simulink model "PI_Level_Control"  (R2024b)
settings: Solver=VariableStepAuto  StartTime=0.0  StopTime=1000  RelTol=1e-3
values from neighbouring files (symbols this model uses):
  C = 6.8    [Arduino_Control_Script.m]    (also in PI_Level_Control_Script.m)
  k = 0.032    [Arduino_Control_Script.m]    (also in PI_Level_Control_Script.m)
  k1 = 0.624    [Arduino_Control_Script.m]    (also in PI_Level_Control_Script.m)
  k11 = k2^2+4*(k-k3)*k1    (= 0.0815946)    [Arduino_Control_Script.m]    (also in PI_Level_Control_Script.m)
  k12 = 8*(k-k3)    (= 0.2608)    [Arduino_Control_Script.m]    (also in PI_Level_Control_Script.m)
  k13 = 2*(k-k3)    (= 0.0652)    [Arduino_Control_Script.m]    (also in PI_Level_Control_Script.m)
  k2 = -0.015    [Arduino_Control_Script.m]    (also in PI_Level_Control_Script.m)
  k3 = -0.0006    [Arduino_Control_Script.m]    (also in PI_Level_Control_Script.m)
  keta = 8*10^-5    (= 8e-05)    [Arduino_Control_Script.m]    (also in PI_Level_Control_Script.m)
libraries: slpidlib x20
(part 2 of 3)

== system PI_Level_Control/Model Proces ==
  ua : Inport
  Amplificator : Subsystem
  Curent Rotoric : Subsystem
  Filtru : Subsystem
  Motor : Subsystem
  Pompa : Subsystem
  Randament Pompa : Subsystem
  Rezervor : Subsystem
  h : Outport
  q : Outport  Port=2
  wires:
  Randament Pompa/1(eta) -> Curent Rotoric/3(eta)
  Rezervor/1(h) -> h/1, Curent Rotoric/1(h), Pompa/2(h)
  Curent Rotoric/1(im) -> Motor/2(im)
  Amplificator/1(um) -> Motor/1(um), Randament Pompa/2(um), Curent Rotoric/4(um)
  ua/1 -> Amplificator/1(ua)
  Filtru/1(q_f) -> Rezervor/1(q), Curent Rotoric/2(q), q/1, Randament Pompa/1(q)
  Pompa/1(q) -> Filtru/1(q)
  Motor/1(kn) -> Pompa/1(kn)

== system PI_Level_Control/Model Proces Nivel ==
  ua : Inport
  Amplificator : Subsystem
  Curent Rotoric : Subsystem
  Filtru : Subsystem
  Motor : Subsystem
  Pompa : Subsystem
  Randament Pompa : Subsystem
  Rezervor : Subsystem
  h : Outport
  q : Outport  Port=2
  wires:
  Randament Pompa/1(eta) -> Curent Rotoric/3(eta)
  Rezervor/1(h) -> h/1, Curent Rotoric/1(h), Pompa/2(h)
  Curent Rotoric/1(im) -> Motor/2(im)
  Amplificator/1(um) -> Motor/1(um), Randament Pompa/2(um), Curent Rotoric/4(um)
  ua/1 -> Amplificator/1(ua)
  Filtru/1(q_f) -> Rezervor/1(q), Curent Rotoric/2(q), q/1, Randament Pompa/1(q)
  Pompa/1(q) -> Filtru/1(q)
  Motor/1(kn) -> Pompa/1(kn)

== system PI_Level_Control/Model Proces Nivel1 ==
  ua : Inport
  Amplificator : Subsystem
  Curent Rotoric : Subsystem
  Filtru : Subsystem
  Motor : Subsystem
  Pompa : Subsystem
  Randament Pompa : Subsystem
  Rezervor : Subsystem
  h : Outport
  q : Outport  Port=2
  wires:
  Randament Pompa/1(eta) -> Curent Rotoric/3(eta)
  Rezervor/1(h) -> h/1, Curent Rotoric/1(h), Pompa/2(h)
  Curent Rotoric/1(im) -> Motor/2(im)
  Amplificator/1(um) -> Motor/1(um), Randament Pompa/2(um), Curent Rotoric/4(um)
  ua/1 -> Amplificator/1(ua)
  Filtru/1(q_f) -> Rezervor/1(q), Curent Rotoric/2(q), q/1, Randament Pompa/1(q)
  Pompa/1(q) -> Filtru/1(q)
  Motor/1(kn) -> Pompa/1(kn)

== system PI_Level_Control/Model Proces Nivel2 ==
  ua : Inport
  Amplificator : Subsystem
  Curent Rotoric : Subsystem
  Filtru : Subsystem
  Motor : Subsystem
  Pompa : Subsystem
  Randament Pompa : Subsystem
  Rezervor : Subsystem
  h : Outport
  q : Outport  Port=2
  wires:
  Randament Pompa/1(eta) -> Curent Rotoric/3(eta)
  Rezervor/1(h) -> h/1, Curent Rotoric/1(h), Pompa/2(h)
  Curent Rotoric/1(im) -> Motor/2(im)
  Amplificator/1(um) -> Motor/1(um), Randament Pompa/2(um), Curent Rotoric/4(um)
  ua/1 -> Amplificator/1(ua)
  Filtru/1(q_f) -> Rezervor/1(q), Curent Rotoric/2(q), q/1, Randament Pompa/1(q)
  Pompa/1(q) -> Filtru/1(q)
  Motor/1(kn) -> Pompa/1(kn)

== system PI_Level_Control/Model Proces Nivel3 ==
  ua : Inport
  Amplificator : Subsystem
  Curent Rotoric : Subsystem
  Filtru : Subsystem
  Motor : Subsystem
  Pompa : Subsystem
  Randament Pompa : Subsystem
  Rezervor : Subsystem
  h : Outport
  q : Outport  Port=2
  wires:
  Randament Pompa/1(eta) -> Curent Rotoric/3(eta)
  Rezervor/1(h) -> h/1, Curent Rotoric/1(h), Pompa/2(h)
  Curent Rotoric/1(im) -> Motor/2(im)
  Amplificator/1(um) -> Motor/1(um), Randament Pompa/2(um), Curent Rotoric/4(um)
  ua/1 -> Amplificator/1(ua)
  Filtru/1(q_f) -> Rezervor/1(q), Curent Rotoric/2(q), q/1, Randament Pompa/1(q)
  Pompa/1(q) -> Filtru/1(q)
  Motor/1(kn) -> Pompa/1(kn)

== system PI_Level_Control/Model Proces1 ==
  ua : Inport
  Amplificator : Subsystem
  Curent Rotoric : Subsystem
  Filtru : Subsystem
  Motor : Subsystem
  Pompa : Subsystem
  Randament Pompa : Subsystem
  Rezervor : Subsystem
  h : Outport
  wires:
  Randament Pompa/1(eta) -> Curent Rotoric/3(eta)
  Rezervor/1(h) -> h/1, Pompa/2(h), Curent Rotoric/1(h)
  Curent Rotoric/1(im) -> Motor/2(im)
  Amplificator/1(um) -> Motor/1(um), Randament Pompa/2(um), Curent Rotoric/4(um)
  ua/1 -> Amplificator/1(ua)
  Filtru/1(q_f) -> Rezervor/1(q), Randament Pompa/1(q), Curent Rotoric/2(q)
  Pompa/1(q) -> Filtru/1(q)
  Motor/1(kn) -> Pompa/1(kn)

== system PI_Level_Control/Model Proces10 ==
  ua : Inport
  Amplificator : Subsystem
  Curent Rotoric : Subsystem
  Filtru : Subsystem
  Motor : Subsystem
  Pompa cu perturbatie reala : Subsystem
  Randament Pompa : Subsystem
  Rezervor : Subsystem
  Step : Step  Time=250  After=0.1*k  SampleTime=0
  h : Outport
  qi : Outport  Port=2
  wires:
  Randament Pompa/1(eta) -> Curent Rotoric/3(eta)
  Rezervor/1(h) -> Pompa cu perturbatie reala/3(h), Curent Rotoric/1(h), h/1
  Curent Rotoric/1(im) -> Motor/2(im)
  Amplificator/1(um) -> Motor/1(um), Randament Pompa/2(um), Curent Rotoric/4(um)
  ua/1 -> Amplificator/1(ua)
  Pompa cu perturbatie reala/1(q) -> Filtru/1(q)
  Motor/1(kn) -> Pompa cu perturbatie reala/1(kn)
  Filtru/1(q_f) -> Rezervor/1(q), Randament Pompa/1(q), qi/1, Curent Rotoric/2(q)
  Step/1 -> Pompa cu perturbatie reala/2(perturbatie k)

== system PI_Level_Control/Model Proces11 ==
  ua : Inport
  Amplificator : Subsystem
  Curent Rotoric : Subsystem
  Filtru : Subsystem
  Motor : Subsystem
  Pompa cu perturbatie reala : Subsystem
  Randament Pompa : Subsystem
  Rezervor1 : Subsystem
  Step : Step  Time=400  After=0.1*k  SampleTime=0
  h : Outport
  qi : Outport  Port=2
  wires:
  Randament Pompa/1(eta) -> Curent Rotoric/3(eta)
  Rezervor1/1(h) -> Pompa cu perturbatie reala/3(h), Curent Rotoric/1(h), h/1
  Curent Rotoric/1(im) -> Motor/2(im)
  Amplificator/1(um) -> Motor/1(um), Randament Pompa/2(um), Curent Rotoric/4(um)
  ua/1 -> Amplificator/1(ua)
  Pompa cu perturbatie reala/1(q) -> Filtru/1(q)
  Motor/1(kn) -> Pompa cu perturbatie reala/1(kn)
  Filtru/1(q_f) -> Rezervor1/1(q), Randament Pompa/1(q), qi/1, Curent Rotoric/2(q)
  Step/1 -> Pompa cu perturbatie reala/2(perturbatie k)

== system PI_Level_Control/Model Proces12 ==
  ua : Inport
  Amplificator : Subsystem
  Curent Rotoric : Subsystem
  Filtru : Subsystem
  Motor : Subsystem
  Pompa cu perturbatie reala : Subsystem
  Randament Pompa : Subsystem
  Rezervor : Subsystem
  perturbatie k : Step  Time=300  After=0.1*k  SampleTime=0
  h : Outport
  qi : Outport  Port=2
  perturbatie : Outport  Port=3
  wires:
  Randament Pompa/1(eta) -> Curent Rotoric/3(eta)
  Rezervor/1(h) -> Pompa cu perturbatie reala/3(h), Curent Rotoric/1(h), h/1
  Curent Rotoric/1(im) -> Motor/2(im)
  Amplificator/1(um) -> Motor/1(um), Randament Pompa/2(um), Curent Rotoric/4(um)
  ua/1 -> Amplificator/1(ua)
  Pompa cu perturbatie reala/1(q) -> Filtru/1(q)
  Motor/1(kn) -> Pompa cu perturbatie reala/1(kn)
  Filtru/1(q_f) -> Randament Pompa/1(q), Curent Rotoric/2(q), qi/1, Rezervor/1(q)
  perturbatie k/1 -> Pompa cu perturbatie reala/2(perturbatie k)
  Rezervor/2(perturbatie) -> perturbatie/1

== system PI_Level_Control/Model Proces13 ==
  ua : Inport
  Amplificator : Subsystem
  Curent Rotoric : Subsystem
  Filtru : Subsystem
  Motor : Subsystem
  Pompa cu perturbatie reala : Subsystem
  Randament Pompa : Subsystem
  Rezervor : Subsystem
  perturbatie k : Step  Time=450  After=0.1*k  SampleTime=0
  h : Outport
  qi : Outport  Port=2
  perturbatie : Outport  Port=3
  wires:
  Randament Pompa/1(eta) -> Curent Rotoric/3(eta)
  Rezervor/1(h) -> Pompa cu perturbatie reala/3(h), Curent Rotoric/1(h), h/1
  Curent Rotoric/1(im) -> Motor/2(im)
  Amplificator/1(um) -> Motor/1(um), Randament Pompa/2(um), Curent Rotoric/4(um)
  ua/1 -> Amplificator/1(ua)
  Pompa cu perturbatie reala/1(q) -> Filtru/1(q)
  Motor/1(kn) -> Pompa cu perturbatie reala/1(kn)
  Filtru/1(q_f) -> Randament Pompa/1(q), Curent Rotoric/2(q), qi/1, Rezervor/1(q)
  perturbatie k/1 -> Pompa cu perturbatie reala/2(perturbatie k)
  Rezervor/2(perturbatie) -> perturbatie/1

== system PI_Level_Control/Model Proces2 ==
  ua : Inport
  Amplificator : Subsystem
  Curent Rotoric : Subsystem
  Filtru : Subsystem
  Motor : Subsystem
  Pompa : Subsystem
  Randament Pompa : Subsystem
  Rezervor : Subsystem
  h : Outport
  wires:
  Randament Pompa/1(eta) -> Curent Rotoric/3(eta)
  Rezervor/1(h) -> h/1, Pompa/2(h), Curent Rotoric/1(h)
  Curent Rotoric/1(im) -> Motor/2(im)
  Amplificator/1(um) -> Motor/1(um), Randament Pompa/2(um), Curent Rotoric/4(um)
  ua/1 -> Amplificator/1(ua)
  Filtru/1(q_f) -> Rezervor/1(q), Randament Pompa/1(q), Curent Rotoric/2(q)
  Pompa/1(q) -> Filtru/1(q)
  Motor/1(kn) -> Pompa/1(kn)

== system PI_Level_Control/Model Proces3 ==
  ua : Inport
  Amplificator : Subsystem
  Curent Rotoric : Subsystem
  Delta qe grafic : Scope
  Detla qe : Display
  Filtru : Subsystem
  Motor : Subsystem
  Pompa : Subsystem
  Randament Pompa : Subsystem
  Rezervor : Subsystem
  h : Outport
  wires:
  Randament Pompa/1(eta) -> Curent Rotoric/3(eta)
  Rezervor/1(h) -> Curent Rotoric/1(h), Pompa/2(h), h/1
  Curent Rotoric/1(im) -> Motor/2(im)
  Amplificator/1(um) -> Motor/1(um), Randament Pompa/2(um), Curent Rotoric/4(um)
  ua/1 -> Amplificator/1(ua)
  Filtru/1(q_f) -> Randament Pompa/1(q), Curent Rotoric/2(q), Rezervor/1(q)
  Pompa/1(q) -> Filtru/1(q)
  Motor/1(kn) -> Pompa/1(kn)
  Rezervor/2(perturbatie) -> Delta qe grafic/1, Detla qe/1

== system PI_Level_Control/Model Proces4 ==
  ua : Inport
  Amplificator : Subsystem
  Curent Rotoric : Subsystem
  Delta qe grafic : Scope
  Detla qe : Display
  Filtru : Subsystem
  Motor : Subsystem
  Pompa : Subsystem
  Randament Pompa : Subsystem
  Rezervor : Subsystem
  h : Outport
  wires:
  Randament Pompa/1(eta) -> Curent Rotoric/3(eta)
  Rezervor/1(h) -> Curent Rotoric/1(h), Pompa/2(h), h/1
  Curent Rotoric/1(im) -> Motor/2(im)
  Amplificator/1(um) -> Motor/1(um), Randament Pompa/2(um), Curent Rotoric/4(um)
  ua/1 -> Amplificator/1(ua)
  Filtru/1(q_f) -> Randament Pompa/1(q), Curent Rotoric/2(q), Rezervor/1(q)
  Pompa/1(q) -> Filtru/1(q)
  Motor/1(kn) -> Pompa/1(kn)
  Rezervor/2(perturbatie) -> Delta qe grafic/1, Detla qe/1

== system PI_Level_Control/Model Proces5 ==
  ua : Inport
  Amplificator : Subsystem
  Curent Rotoric : Subsystem
  Filtru : Subsystem
  Motor : Subsystem
  Perturbatie 10%k : Step  Time=250  After=k*0.1  SampleTime=0
  Pompa cu perturbatie reala : Subsystem
  Randament Pompa : Subsystem
  Rezervor : Subsystem
  h : Outport
  wires:
  Randament Pompa/1(eta) -> Curent Rotoric/3(eta)
  Rezervor/1(h) -> h/1, Pompa cu perturbatie reala/3(h), Curent Rotoric/1(h)
  Curent Rotoric/1(im) -> Motor/2(im)
  Amplificator/1(um) -> Motor/1(um), Randament Pompa/2(um), Curent Rotoric/4(um)
  ua/1 -> Amplificator/1(ua)
  Filtru/1(q_f) -> Rezervor/1(q), Randament Pompa/1(q), Curent Rotoric/2(q)
  Pompa cu perturbatie reala/1(q) -> Filtru/1(q)
  Motor/1(kn) -> Pompa cu perturbatie reala/1(kn)
  Perturbatie 10%k/1 -> Pompa cu perturbatie reala/2(perturbatie k)

== system PI_Level_Control/Model Proces6 ==
  ua : Inport
  Amplificator : Subsystem
  Curent Rotoric : Subsystem
  Filtru : Subsystem
  Motor : Subsystem
  Perturbatie 10%k : Step  Time=250  After=k*0.1  SampleTime=0
  Pompa cu perturbatie reala : Subsystem
  Randament Pompa : Subsystem
  Rezervor1 : Subsystem
  h : Outport
  wires:
  Randament Pompa/1(eta) -> Curent Rotoric/3(eta)
  Rezervor1/1(h) -> h/1, Pompa cu perturbatie reala/3(h), Curent Rotoric/1(h)
  Curent Rotoric/1(im) -> Motor/2(im)
  Amplificator/1(um) -> Motor/1(um), Randament Pompa/2(um), Curent Rotoric/4(um)
  ua/1 -> Amplificator/1(ua)
  Filtru/1(q_f) -> Rezervor1/1(q), Randament Pompa/1(q), Curent Rotoric/2(q)
  Pompa cu perturbatie reala/1(q) -> Filtru/1(q)
  Motor/1(kn) -> Pompa cu perturbatie reala/1(kn)
  Perturbatie 10%k/1 -> Pompa cu perturbatie reala/2(perturbatie k)

== system PI_Level_Control/Model Proces7 ==
  ua : Inport
  Amplificator : Subsystem
  Curent Rotoric : Subsystem
  Filtru : Subsystem
  Motor : Subsystem
  Pompa : Subsystem
  Randament Pompa : Subsystem
  Rezervor : Subsystem
  h : Outport
  perturbatie delta qe : Outport  Port=2
  wires:
  Randament Pompa/1(eta) -> Curent Rotoric/3(eta)
  Rezervor/1(h) -> Curent Rotoric/1(h), Pompa/2(h), h/1
  Curent Rotoric/1(im) -> Motor/2(im)
  Amplificator/1(um) -> Motor/1(um), Randament Pompa/2(um), Curent Rotoric/4(um)
  ua/1 -> Amplificator/1(ua)
  Filtru/1(q_f) -> Randament Pompa/1(q), Curent Rotoric/2(q), Rezervor/1(q)
  Pompa/1(q) -> Filtru/1(q)
  Motor/1(kn) -> Pompa/1(kn)
  Rezervor/2(perturbatie) -> perturbatie delta qe/1

== system PI_Level_Control/Model Proces8 ==
  ua : Inport
  Amplificator : Subsystem
  Curent Rotoric : Subsystem
  Filtru : Subsystem
  Motor : Subsystem
  Pompa : Subsystem
  Randament Pompa : Subsystem
  Rezervor : Subsystem
  h : Outport
  perturbatie delta qe : Outport  Port=2
  wires:
  Randament Pompa/1(eta) -> Curent Rotoric/3(eta)
  Rezervor/1(h) -> Curent Rotoric/1(h), Pompa/2(h), h/1
  Curent Rotoric/1(im) -> Motor/2(im)
  Amplificator/1(um) -> Motor/1(um), Randament Pompa/2(um), Curent Rotoric/4(um)
  ua/1 -> Amplificator/1(ua)
  Filtru/1(q_f) -> Randament Pompa/1(q), Curent Rotoric/2(q), Rezervor/1(q)
  Pompa/1(q) -> Filtru/1(q)
  Motor/1(kn) -> Pompa/1(kn)
  Rezervor/2(perturbatie) -> perturbatie delta qe/1

== system PI_Level_Control/Model Proces9 ==
  ua : Inport
  Amplificator : Subsystem
  Curent Rotoric : Subsystem
  Filtru : Subsystem
  Motor : Subsystem
  Pompa : Subsystem
  Randament Pompa : Subsystem
  Rezervor : Subsystem
  h : Outport
  qi : Outport  Port=2
  wires:
  Randament Pompa/1(eta) -> Curent Rotoric/3(eta)
  Rezervor/1(h) -> Curent Rotoric/1(h), Pompa/2(h), h/1
  Curent Rotoric/1(im) -> Motor/2(im)
  Amplificator/1(um) -> Motor/1(um), Randament Pompa/2(um), Curent Rotoric/4(um)
  ua/1 -> Amplificator/1(ua)
  Pompa/1(q) -> Filtru/1(q)
  Motor/1(kn) -> Pompa/1(kn)
  Filtru/1(q_f) -> qi/1, Randament Pompa/1(q), Curent Rotoric/2(q), Rezervor/1(q)

== system PI_Level_Control/Model Proces/Amplificator ==
  ua : Inport
  Constant : Constant  Value=8.1
  Gain : Gain  Gain=2.2
  Gain1 : Gain  Gain=2.2
  Gain2 : Gain  Gain=5
  Saturation : Saturate  UpperLimit=22  LowerLimit=0
  Sum : Sum  Inputs=|+-
  Sum1 : Sum  Inputs=|++
  Switch : Switch  Threshold=8.1  SaturateOnIntegerOverflow=off  InputSameDT=off
  um : Outport
  wires:
  ua/1 -> Gain/1, Sum/1, Gain1/1, Switch/2
  Gain1/1 -> Sum1/1
  Gain/1 -> Switch/3
  Sum1/1 -> Switch/1
  Gain2/1 -> Sum1/2
  Constant/1 -> Sum/2
  Switch/1 -> Saturation/1
  Sum/1 -> Gain2/1
  Saturation/1 -> um/1

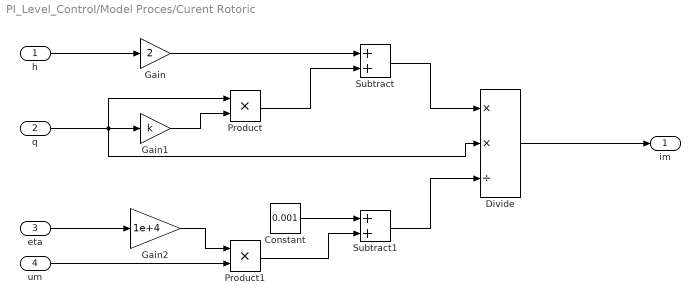
== system PI_Level_Control/Model Proces/Curent Rotoric ==
  h : Inport
  q : Inport  Port=2
  eta : Inport  Port=3
  um : Inport  Port=4
  Constant : Constant  Value=0.001
  Divide : Product  Inputs=**/
  Gain : Gain  Gain=2
  Gain1 : Gain  Gain=k
  Gain2 : Gain  Gain=1e+4
  Product : Product
  Product1 : Product
  Subtract : Sum
  Subtract1 : Sum
  im : Outport
  wires:
  Divide/1 -> im/1
  Subtract1/1 -> Divide/3
  Constant/1 -> Subtract1/1
  Gain2/1 -> Product1/1
  q/1 -> Divide/2, Product/1, Gain1/1
  Subtract/1 -> Divide/1
  Product/1 -> Subtract/2
  Gain/1 -> Subtract/1
  Gain1/1 -> Product/2
  Product1/1 -> Subtract1/2
  um/1 -> Product1/2
  h/1 -> Gain/1
  eta/1 -> Gain2/1

== system PI_Level_Control/Model Proces/Filtru ==
  q : Inport
  Integrator : Integrator  InitialCondition=29.18
  Sum : Sum  Inputs=|+-
  q_f : Outport
  wires:
  Sum/1 -> Integrator/1
  Integrator/1 -> q_f/1, Sum/2
  q/1 -> Sum/1

== system PI_Level_Control/Model Proces/Motor ==
  um : Inport
  im : Inport  Port=2
  Add : Sum  Inputs=+-
  Rm : Gain  Gain=3
  kn : Outport
  wires:
  Rm/1 -> Add/2
  um/1 -> Add/1
  im/1 -> Rm/1
  Add/1 -> kn/1

== system PI_Level_Control/Model Proces/Pompa ==
  kn : Inport
  h : Inport  Port=2
  Gain : Gain  Gain=k2
  Gain1 : Gain  Gain=k11
  Gain2 : Gain  Gain=k12
  Gain3 : Gain  Gain=1/k13
  Product : Product
  Sqrt : Sqrt
  Subtract : Sum  Inputs=+-
  Subtract1 : Sum
  q : Outport
  wires:
  Gain1/1 -> Subtract/1
  Gain2/1 -> Subtract/2
  Product/1 -> Gain1/1
  Gain/1 -> Subtract1/1
  kn/1 -> Product/2, Product/1, Gain/1
  Subtract/1 -> Sqrt/1
  Subtract1/1 -> Gain3/1
  Sqrt/1 -> Subtract1/2
  Gain3/1 -> q/1
  h/1 -> Gain2/1

== system PI_Level_Control/Model Proces/Randament Pompa ==
  q : Inport
  um : Inport  Port=2
  Gain : Gain  Gain=keta
  Product : Product
  eta : Outport
  wires:
  Gain/1 -> Product/2
  Product/1 -> eta/1
  q/1 -> Product/1
  um/1 -> Gain/1

== system PI_Level_Control/Model Proces/Rezervor ==
  q : Inport
  Fcn : Fcn  Expr=sqrt(u)*9
  Gain : Gain  Gain=1/332.5
  Integrator : Integrator  InitialCondition=10.51
  Sum : Sum  Inputs=|+-
  h : Outport
  wires:
  Gain/1 -> Integrator/1
  Fcn/1 -> Sum/2
  Integrator/1 -> h/1, Fcn/1
  Sum/1 -> Gain/1
  q/1 -> Sum/1

== system PI_Level_Control/Model Proces Nivel/Amplificator ==
  ua : Inport
  Constant : Constant  Value=8.1
  Gain : Gain  Gain=2.2
  Gain1 : Gain  Gain=2.2
  Gain2 : Gain  Gain=5
  Saturation : Saturate  UpperLimit=22  LowerLimit=0
  Sum : Sum  Inputs=|+-
  Sum1 : Sum  Inputs=|++
  Switch : Switch  Threshold=8.1  SaturateOnIntegerOverflow=off  InputSameDT=off
  um : Outport
  wires:
  ua/1 -> Gain/1, Sum/1, Gain1/1, Switch/2
  Gain1/1 -> Sum1/1
  Gain/1 -> Switch/3
  Sum1/1 -> Switch/1
  Gain2/1 -> Sum1/2
  Constant/1 -> Sum/2
  Switch/1 -> Saturation/1
  Sum/1 -> Gain2/1
  Saturation/1 -> um/1

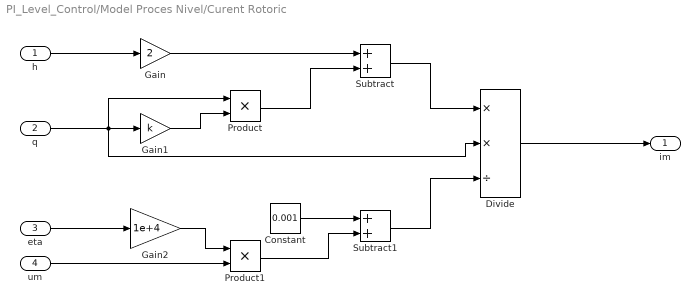
== system PI_Level_Control/Model Proces Nivel/Curent Rotoric ==
  h : Inport
  q : Inport  Port=2
  eta : Inport  Port=3
  um : Inport  Port=4
  Constant : Constant  Value=0.001
  Divide : Product  Inputs=**/
  Gain : Gain  Gain=2
  Gain1 : Gain  Gain=k
  Gain2 : Gain  Gain=1e+4
  Product : Product
  Product1 : Product
  Subtract : Sum
  Subtract1 : Sum
  im : Outport
  wires:
  Divide/1 -> im/1
  Subtract1/1 -> Divide/3
  Constant/1 -> Subtract1/1
  Gain2/1 -> Product1/1
  q/1 -> Divide/2, Product/1, Gain1/1
  Subtract/1 -> Divide/1
  Product/1 -> Subtract/2
  Gain/1 -> Subtract/1
  Gain1/1 -> Product/2
  Product1/1 -> Subtract1/2
  um/1 -> Product1/2
  h/1 -> Gain/1
  eta/1 -> Gain2/1

== system PI_Level_Control/Model Proces Nivel/Filtru ==
  q : Inport
  Integrator : Integrator  InitialCondition=27.3
  Sum : Sum  Inputs=|+-
  q_f : Outport
  wires:
  Sum/1 -> Integrator/1
  Integrator/1 -> q_f/1, Sum/2
  q/1 -> Sum/1

== system PI_Level_Control/Model Proces Nivel/Motor ==
  um : Inport
  im : Inport  Port=2
  Add : Sum  Inputs=+-
  Rm : Gain  Gain=3
  kn : Outport
  wires:
  Rm/1 -> Add/2
  um/1 -> Add/1
  im/1 -> Rm/1
  Add/1 -> kn/1

== system PI_Level_Control/Model Proces Nivel/Pompa ==
  kn : Inport
  h : Inport  Port=2
  Gain : Gain  Gain=k2
  Gain1 : Gain  Gain=k11
  Gain2 : Gain  Gain=k12
  Gain3 : Gain  Gain=1/k13
  Product : Product
  Sqrt : Sqrt
  Subtract : Sum  Inputs=+-
  Subtract1 : Sum
  q : Outport
  wires:
  Gain1/1 -> Subtract/1
  Gain2/1 -> Subtract/2
  Product/1 -> Gain1/1
  Gain/1 -> Subtract1/1
  kn/1 -> Product/2, Product/1, Gain/1
  Subtract/1 -> Sqrt/1
  Subtract1/1 -> Gain3/1
  Sqrt/1 -> Subtract1/2
  Gain3/1 -> q/1
  h/1 -> Gain2/1

== system PI_Level_Control/Model Proces Nivel/Randament Pompa ==
  q : Inport
  um : Inport  Port=2
  Gain : Gain  Gain=keta
  Product : Product
  eta : Outport
  wires:
  Gain/1 -> Product/2
  Product/1 -> eta/1
  q/1 -> Product/1
  um/1 -> Gain/1

== system PI_Level_Control/Model Proces Nivel/Rezervor ==
  q : Inport
  Fcn : Fcn  Expr=sqrt(u)*6.8
  Gain : Gain  Gain=1/332.5
  Integrator : Integrator  InitialCondition=16.02
  Sum : Sum  Inputs=|+-
  h : Outport
  wires:
  Gain/1 -> Integrator/1
  Fcn/1 -> Sum/2
  Integrator/1 -> h/1, Fcn/1
  Sum/1 -> Gain/1
  q/1 -> Sum/1

== system PI_Level_Control/Model Proces Nivel1/Amplificator ==
  ua : Inport
  Constant : Constant  Value=8.1
  Gain : Gain  Gain=2.2
  Gain1 : Gain  Gain=2.2
  Gain2 : Gain  Gain=5
  Saturation : Saturate  UpperLimit=22  LowerLimit=0
  Sum : Sum  Inputs=|+-
  Sum1 : Sum  Inputs=|++
  Switch : Switch  Threshold=8.1  SaturateOnIntegerOverflow=off  InputSameDT=off
  um : Outport
  wires:
  ua/1 -> Gain/1, Sum/1, Gain1/1, Switch/2
  Gain1/1 -> Sum1/1
  Gain/1 -> Switch/3
  Sum1/1 -> Switch/1
  Gain2/1 -> Sum1/2
  Constant/1 -> Sum/2
  Switch/1 -> Saturation/1
  Sum/1 -> Gain2/1
  Saturation/1 -> um/1

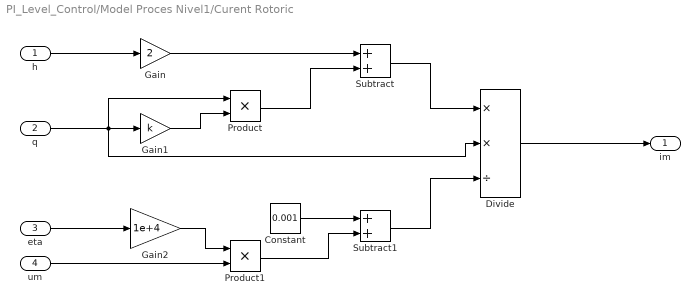
== system PI_Level_Control/Model Proces Nivel1/Curent Rotoric ==
  h : Inport
  q : Inport  Port=2
  eta : Inport  Port=3
  um : Inport  Port=4
  Constant : Constant  Value=0.001
  Divide : Product  Inputs=**/
  Gain : Gain  Gain=2
  Gain1 : Gain  Gain=k
  Gain2 : Gain  Gain=1e+4
  Product : Product
  Product1 : Product
  Subtract : Sum
  Subtract1 : Sum
  im : Outport
  wires:
  Divide/1 -> im/1
  Subtract1/1 -> Divide/3
  Constant/1 -> Subtract1/1
  Gain2/1 -> Product1/1
  q/1 -> Divide/2, Product/1, Gain1/1
  Subtract/1 -> Divide/1
  Product/1 -> Subtract/2
  Gain/1 -> Subtract/1
  Gain1/1 -> Product/2
  Product1/1 -> Subtract1/2
  um/1 -> Product1/2
  h/1 -> Gain/1
  eta/1 -> Gain2/1

== system PI_Level_Control/Model Proces Nivel1/Filtru ==
  q : Inport
  Integrator : Integrator  InitialCondition=27.3
  Sum : Sum  Inputs=|+-
  q_f : Outport
  wires:
  Sum/1 -> Integrator/1
  Integrator/1 -> q_f/1, Sum/2
  q/1 -> Sum/1

== system PI_Level_Control/Model Proces Nivel1/Motor ==
  um : Inport
  im : Inport  Port=2
  Add : Sum  Inputs=+-
  Rm : Gain  Gain=3
  kn : Outport
  wires:
  Rm/1 -> Add/2
  um/1 -> Add/1
  im/1 -> Rm/1
  Add/1 -> kn/1

== system PI_Level_Control/Model Proces Nivel1/Pompa ==
  kn : Inport
  h : Inport  Port=2
  Gain : Gain  Gain=k2
  Gain1 : Gain  Gain=k11
  Gain2 : Gain  Gain=k12
  Gain3 : Gain  Gain=1/k13
  Product : Product
  Sqrt : Sqrt
  Subtract : Sum  Inputs=+-
  Subtract1 : Sum
  q : Outport
  wires:
  Gain1/1 -> Subtract/1
  Gain2/1 -> Subtract/2
  Product/1 -> Gain1/1
  Gain/1 -> Subtract1/1
  kn/1 -> Product/2, Product/1, Gain/1
  Subtract/1 -> Sqrt/1
  Subtract1/1 -> Gain3/1
  Sqrt/1 -> Subtract1/2
  Gain3/1 -> q/1
  h/1 -> Gain2/1

== system PI_Level_Control/Model Proces Nivel1/Randament Pompa ==
  q : Inport
  um : Inport  Port=2
  Gain : Gain  Gain=keta
  Product : Product
  eta : Outport
  wires:
  Gain/1 -> Product/2
  Product/1 -> eta/1
  q/1 -> Product/1
  um/1 -> Gain/1

== system PI_Level_Control/Model Proces Nivel1/Rezervor ==
  q : Inport
  Fcn : Fcn  Expr=sqrt(u)*6.8
  Gain : Gain  Gain=1/332.5
  Integrator : Integrator  InitialCondition=16.02
  Sum : Sum  Inputs=|+-
  h : Outport
  wires:
  Gain/1 -> Integrator/1
  Fcn/1 -> Sum/2
  Integrator/1 -> h/1, Fcn/1
  Sum/1 -> Gain/1
  q/1 -> Sum/1

== system PI_Level_Control/Model Proces Nivel2/Amplificator ==
  ua : Inport
  Constant : Constant  Value=8.1
  Gain : Gain  Gain=2.2
  Gain1 : Gain  Gain=2.2
  Gain2 : Gain  Gain=5
  Saturation : Saturate  UpperLimit=22  LowerLimit=0
  Sum : Sum  Inputs=|+-
  Sum1 : Sum  Inputs=|++
  Switch : Switch  Threshold=8.1  SaturateOnIntegerOverflow=off  InputSameDT=off
  um : Outport
  wires:
  ua/1 -> Gain/1, Sum/1, Gain1/1, Switch/2
  Gain1/1 -> Sum1/1
  Gain/1 -> Switch/3
  Sum1/1 -> Switch/1
  Gain2/1 -> Sum1/2
  Constant/1 -> Sum/2
  Switch/1 -> Saturation/1
  Sum/1 -> Gain2/1
  Saturation/1 -> um/1

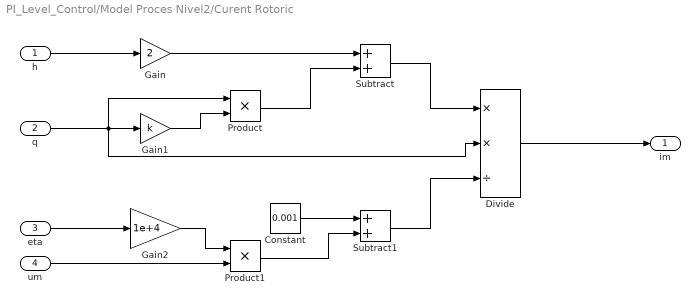
== system PI_Level_Control/Model Proces Nivel2/Curent Rotoric ==
  h : Inport
  q : Inport  Port=2
  eta : Inport  Port=3
  um : Inport  Port=4
  Constant : Constant  Value=0.001
  Divide : Product  Inputs=**/
  Gain : Gain  Gain=2
  Gain1 : Gain  Gain=k
  Gain2 : Gain  Gain=1e+4
  Product : Product
  Product1 : Product
  Subtract : Sum
  Subtract1 : Sum
  im : Outport
  wires:
  Divide/1 -> im/1
  Subtract1/1 -> Divide/3
  Constant/1 -> Subtract1/1
  Gain2/1 -> Product1/1
  q/1 -> Divide/2, Product/1, Gain1/1
  Subtract/1 -> Divide/1
  Product/1 -> Subtract/2
  Gain/1 -> Subtract/1
  Gain1/1 -> Product/2
  Product1/1 -> Subtract1/2
  um/1 -> Product1/2
  h/1 -> Gain/1
  eta/1 -> Gain2/1

== system PI_Level_Control/Model Proces Nivel2/Filtru ==
  q : Inport
  Integrator : Integrator  InitialCondition=27.3
  Sum : Sum  Inputs=|+-
  q_f : Outport
  wires:
  Sum/1 -> Integrator/1
  Integrator/1 -> q_f/1, Sum/2
  q/1 -> Sum/1

== system PI_Level_Control/Model Proces Nivel2/Motor ==
  um : Inport
  im : Inport  Port=2
  Add : Sum  Inputs=+-
  Rm : Gain  Gain=3
  kn : Outport
  wires:
  Rm/1 -> Add/2
  um/1 -> Add/1
  im/1 -> Rm/1
  Add/1 -> kn/1

== system PI_Level_Control/Model Proces Nivel2/Pompa ==
  kn : Inport
  h : Inport  Port=2
  Gain : Gain  Gain=k2
  Gain1 : Gain  Gain=k11
  Gain2 : Gain  Gain=k12
  Gain3 : Gain  Gain=1/k13
  Product : Product
  Sqrt : Sqrt
  Subtract : Sum  Inputs=+-
  Subtract1 : Sum
  q : Outport
  wires:
  Gain1/1 -> Subtract/1
  Gain2/1 -> Subtract/2
  Product/1 -> Gain1/1
  Gain/1 -> Subtract1/1
  kn/1 -> Product/2, Product/1, Gain/1
  Subtract/1 -> Sqrt/1
  Subtract1/1 -> Gain3/1
  Sqrt/1 -> Subtract1/2
  Gain3/1 -> q/1
  h/1 -> Gain2/1

== system PI_Level_Control/Model Proces Nivel2/Randament Pompa ==
  q : Inport
  um : Inport  Port=2
  Gain : Gain  Gain=keta
  Product : Product
  eta : Outport
  wires:
  Gain/1 -> Product/2
  Product/1 -> eta/1
  q/1 -> Product/1
  um/1 -> Gain/1

== system PI_Level_Control/Model Proces Nivel2/Rezervor ==
  q : Inport
  Fcn : Fcn  Expr=sqrt(u)*6.8
  Gain : Gain  Gain=1/332.5
  Integrator : Integrator  InitialCondition=16.02
  Sum : Sum  Inputs=|+-
  h : Outport
  wires:
  Gain/1 -> Integrator/1
  Fcn/1 -> Sum/2
  Integrator/1 -> h/1, Fcn/1
  Sum/1 -> Gain/1
  q/1 -> Sum/1

== system PI_Level_Control/Model Proces Nivel3/Amplificator ==
  ua : Inport
  Constant : Constant  Value=8.1
  Gain : Gain  Gain=2.2
  Gain1 : Gain  Gain=2.2
  Gain2 : Gain  Gain=5
  Saturation : Saturate  UpperLimit=22  LowerLimit=0
  Sum : Sum  Inputs=|+-
  Sum1 : Sum  Inputs=|++
  Switch : Switch  Threshold=8.1  SaturateOnIntegerOverflow=off  InputSameDT=off
  um : Outport
  wires:
  ua/1 -> Gain/1, Sum/1, Gain1/1, Switch/2
  Gain1/1 -> Sum1/1
  Gain/1 -> Switch/3
  Sum1/1 -> Switch/1
  Gain2/1 -> Sum1/2
  Constant/1 -> Sum/2
  Switch/1 -> Saturation/1
  Sum/1 -> Gain2/1
  Saturation/1 -> um/1

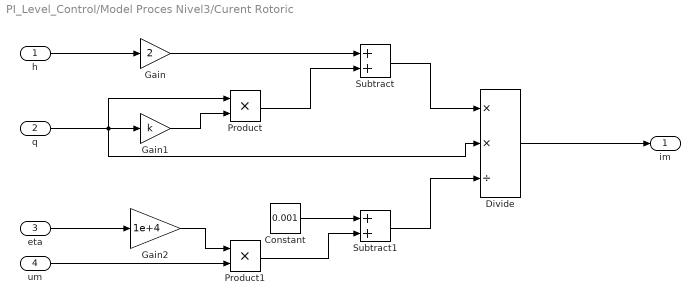
== system PI_Level_Control/Model Proces Nivel3/Curent Rotoric ==
  h : Inport
  q : Inport  Port=2
  eta : Inport  Port=3
  um : Inport  Port=4
  Constant : Constant  Value=0.001
  Divide : Product  Inputs=**/
  Gain : Gain  Gain=2
  Gain1 : Gain  Gain=k
  Gain2 : Gain  Gain=1e+4
  Product : Product
  Product1 : Product
  Subtract : Sum
  Subtract1 : Sum
  im : Outport
  wires:
  Divide/1 -> im/1
  Subtract1/1 -> Divide/3
  Constant/1 -> Subtract1/1
  Gain2/1 -> Product1/1
  q/1 -> Divide/2, Product/1, Gain1/1
  Subtract/1 -> Divide/1
  Product/1 -> Subtract/2
  Gain/1 -> Subtract/1
  Gain1/1 -> Product/2
  Product1/1 -> Subtract1/2
  um/1 -> Product1/2
  h/1 -> Gain/1
  eta/1 -> Gain2/1

== system PI_Level_Control/Model Proces Nivel3/Filtru ==
  q : Inport
  Integrator : Integrator  InitialCondition=27.3
  Sum : Sum  Inputs=|+-
  q_f : Outport
  wires:
  Sum/1 -> Integrator/1
  Integrator/1 -> q_f/1, Sum/2
  q/1 -> Sum/1

== system PI_Level_Control/Model Proces Nivel3/Motor ==
  um : Inport
  im : Inport  Port=2
  Add : Sum  Inputs=+-
  Rm : Gain  Gain=3
  kn : Outport
  wires:
  Rm/1 -> Add/2
  um/1 -> Add/1
  im/1 -> Rm/1
  Add/1 -> kn/1

== system PI_Level_Control/Model Proces Nivel3/Pompa ==
  kn : Inport
  h : Inport  Port=2
  Gain : Gain  Gain=k2
  Gain1 : Gain  Gain=k11
  Gain2 : Gain  Gain=k12
  Gain3 : Gain  Gain=1/k13
  Product : Product
  Sqrt : Sqrt
  Subtract : Sum  Inputs=+-
  Subtract1 : Sum
  q : Outport
  wires:
  Gain1/1 -> Subtract/1
  Gain2/1 -> Subtract/2
  Product/1 -> Gain1/1
  Gain/1 -> Subtract1/1
  kn/1 -> Product/2, Product/1, Gain/1
  Subtract/1 -> Sqrt/1
  Subtract1/1 -> Gain3/1
  Sqrt/1 -> Subtract1/2
  Gain3/1 -> q/1
  h/1 -> Gain2/1

== system PI_Level_Control/Model Proces Nivel3/Randament Pompa ==
  q : Inport
  um : Inport  Port=2
  Gain : Gain  Gain=keta
  Product : Product
  eta : Outport
  wires:
  Gain/1 -> Product/2
  Product/1 -> eta/1
  q/1 -> Product/1
  um/1 -> Gain/1

== system PI_Level_Control/Model Proces Nivel3/Rezervor ==
  q : Inport
  Fcn : Fcn  Expr=sqrt(u)*6.8
  Gain : Gain  Gain=1/332.5
  Integrator : Integrator  InitialCondition=16.02
  Sum : Sum  Inputs=|+-
  h : Outport
  wires:
  Gain/1 -> Integrator/1
  Fcn/1 -> Sum/2
  Integrator/1 -> h/1, Fcn/1
  Sum/1 -> Gain/1
  q/1 -> Sum/1

== system PI_Level_Control/Model Proces1/Amplificator ==
  ua : Inport
  Constant : Constant  Value=8.1
  Gain : Gain  Gain=2.2
  Gain1 : Gain  Gain=2.2
  Gain2 : Gain  Gain=5
  Saturation : Saturate  UpperLimit=22  LowerLimit=0
  Sum : Sum  Inputs=|+-
  Sum1 : Sum  Inputs=|++
  Switch : Switch  Threshold=8.1  SaturateOnIntegerOverflow=off  InputSameDT=off
  um : Outport
  wires:
  ua/1 -> Gain/1, Sum/1, Gain1/1, Switch/2
  Gain1/1 -> Sum1/1
  Gain/1 -> Switch/3
  Sum1/1 -> Switch/1
  Gain2/1 -> Sum1/2
  Constant/1 -> Sum/2
  Switch/1 -> Saturation/1
  Sum/1 -> Gain2/1
  Saturation/1 -> um/1

== system PI_Level_Control/Model Proces1/Curent Rotoric ==
  h : Inport
  q : Inport  Port=2
  eta : Inport  Port=3
  um : Inport  Port=4
  Constant : Constant  Value=000.1
  Divide : Product  Inputs=**/
  Gain : Gain  Gain=2
  Gain1 : Gain  Gain=k
  Gain2 : Gain  Gain=1e+4
  Product : Product
  Product1 : Product
  Subtract : Sum
  Subtract1 : Sum
  im : Outport
  wires:
  Divide/1 -> im/1
  Subtract1/1 -> Divide/3
  Constant/1 -> Subtract1/1
  Gain2/1 -> Product1/1
  q/1 -> Divide/2, Product/1, Gain1/1
  Subtract/1 -> Divide/1
  Product/1 -> Subtract/2
  Gain/1 -> Subtract/1
  Gain1/1 -> Product/2
  Product1/1 -> Subtract1/2
  um/1 -> Product1/2
  h/1 -> Gain/1
  eta/1 -> Gain2/1

== system PI_Level_Control/Model Proces1/Filtru ==
  q : Inport
  Integrator : Integrator  InitialCondition=29.2
  Sum : Sum  Inputs=|+-
  q_f : Outport
  wires:
  Sum/1 -> Integrator/1
  Integrator/1 -> q_f/1, Sum/2
  q/1 -> Sum/1

== system PI_Level_Control/Model Proces1/Motor ==
  um : Inport
  im : Inport  Port=2
  Add : Sum  Inputs=+-
  Rm : Gain  Gain=3
  kn : Outport
  wires:
  Rm/1 -> Add/2
  um/1 -> Add/1
  im/1 -> Rm/1
  Add/1 -> kn/1

== system PI_Level_Control/Model Proces1/Pompa ==
  kn : Inport
  h : Inport  Port=2
  Gain : Gain  Gain=k2
  Gain1 : Gain  Gain=k11
  Gain2 : Gain  Gain=k12
  Gain3 : Gain  Gain=1/k13
  Product : Product
  Sqrt : Sqrt
  Subtract : Sum  Inputs=+-
  Subtract1 : Sum
  q : Outport
  wires:
  Gain1/1 -> Subtract/1
  Gain2/1 -> Subtract/2
  Product/1 -> Gain1/1
  Gain/1 -> Subtract1/1
  kn/1 -> Product/2, Product/1, Gain/1
  Subtract/1 -> Sqrt/1
  Subtract1/1 -> Gain3/1
  Sqrt/1 -> Subtract1/2
  Gain3/1 -> q/1
  h/1 -> Gain2/1

== system PI_Level_Control/Model Proces1/Randament Pompa ==
  q : Inport
  um : Inport  Port=2
  Gain : Gain  Gain=keta
  Product : Product
  eta : Outport
  wires:
  Gain/1 -> Product/2
  Product/1 -> eta/1
  q/1 -> Product/1
  um/1 -> Gain/1

== system PI_Level_Control/Model Proces1/Rezervor ==
  q : Inport
  Fcn : Fcn  Expr=sqrt(u)*9
  Gain : Gain  Gain=1/332.5
  Integrator : Integrator  InitialCondition=10.51
  Sum : Sum  Inputs=|+-
  h : Outport
  wires:
  Gain/1 -> Integrator/1
  Fcn/1 -> Sum/2
  Integrator/1 -> h/1, Fcn/1
  Sum/1 -> Gain/1
  q/1 -> Sum/1

== system PI_Level_Control/Model Proces10/Amplificator ==
  ua : Inport
  Constant : Constant  Value=8.1
  Gain : Gain  Gain=2.2
  Gain1 : Gain  Gain=2.2
  Gain2 : Gain  Gain=5
  Saturation : Saturate  UpperLimit=22  LowerLimit=0
  Sum : Sum  Inputs=|+-
  Sum1 : Sum  Inputs=|++
  Switch : Switch  Threshold=8.1  SaturateOnIntegerOverflow=off  InputSameDT=off
  um : Outport
  wires:
  ua/1 -> Gain/1, Sum/1, Gain1/1, Switch/2
  Gain1/1 -> Sum1/1
  Gain/1 -> Switch/3
  Sum1/1 -> Switch/1
  Gain2/1 -> Sum1/2
  Constant/1 -> Sum/2
  Switch/1 -> Saturation/1
  Sum/1 -> Gain2/1
  Saturation/1 -> um/1

== system PI_Level_Control/Model Proces10/Curent Rotoric ==
  h : Inport
  q : Inport  Port=2
  eta : Inport  Port=3
  um : Inport  Port=4
  Constant : Constant  Value=000.1
  Divide : Product  Inputs=**/
  Gain : Gain  Gain=2
  Gain1 : Gain  Gain=k
  Gain2 : Gain  Gain=1e+4
  Product : Product
  Product1 : Product
  Subtract : Sum
  Subtract1 : Sum
  im : Outport
  wires:
  Divide/1 -> im/1
  Subtract1/1 -> Divide/3
  Constant/1 -> Subtract1/1
  Gain2/1 -> Product1/1
  q/1 -> Divide/2, Product/1, Gain1/1
  Subtract/1 -> Divide/1
  Product/1 -> Subtract/2
  Gain/1 -> Subtract/1
  Gain1/1 -> Product/2
  Product1/1 -> Subtract1/2
  um/1 -> Product1/2
  h/1 -> Gain/1
  eta/1 -> Gain2/1

== system PI_Level_Control/Model Proces10/Filtru ==
  q : Inport
  Integrator : Integrator  InitialCondition=29.18
  Sum : Sum  Inputs=|+-
  q_f : Outport
  wires:
  Sum/1 -> Integrator/1
  Integrator/1 -> q_f/1, Sum/2
  q/1 -> Sum/1

== system PI_Level_Control/Model Proces10/Motor ==
  um : Inport
  im : Inport  Port=2
  Add : Sum  Inputs=+-
  Rm : Gain  Gain=3
  kn : Outport
  wires:
  Rm/1 -> Add/2
  um/1 -> Add/1
  im/1 -> Rm/1
  Add/1 -> kn/1

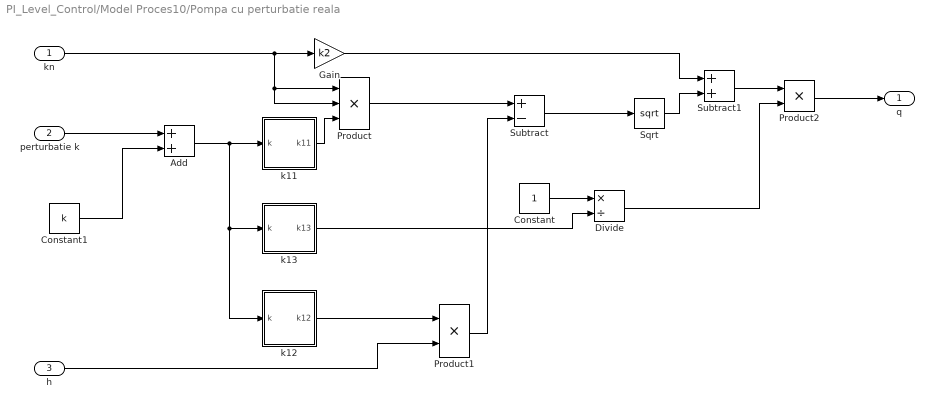
== system PI_Level_Control/Model Proces10/Pompa cu perturbatie reala ==
  kn : Inport
  perturbatie k : Inport  Port=2
  h : Inport  Port=3
  Add : Sum
  Constant : Constant
  Constant1 : Constant  Value=k
  Divide : Product  Inputs=*/
  Gain : Gain  Gain=k2
  Product : Product  Inputs=3
  Product1 : Product
  Product2 : Product
  Sqrt : Sqrt
  Subtract : Sum  Inputs=+-
  Subtract1 : Sum
  k11 : Subsystem
  k12 : Subsystem
  k13 : Subsystem
  q : Outport
  wires:
  h/1 -> Product1/2
  k12/1(k12) -> Product1/1
  Constant1/1 -> Add/2
  Add/1 -> k12/1(k), k13/1(k), k11/1(k)
  Gain/1 -> Subtract1/1
  Product/1 -> Subtract/1
  Divide/1 -> Product2/2
  kn/1 -> Product/2, Product/1, Gain/1
  Subtract/1 -> Sqrt/1
  k13/1(k13) -> Divide/2
  Subtract1/1 -> Product2/1
  k11/1(k11) -> Product/3
  Constant/1 -> Divide/1
  Product1/1 -> Subtract/2
  Sqrt/1 -> Subtract1/2
  perturbatie k/1 -> Add/1
  Product2/1 -> q/1

== system PI_Level_Control/Model Proces10/Randament Pompa ==
  q : Inport
  um : Inport  Port=2
  Gain : Gain  Gain=keta
  Product : Product
  eta : Outport
  wires:
  Gain/1 -> Product/2
  Product/1 -> eta/1
  q/1 -> Product/1
  um/1 -> Gain/1

== system PI_Level_Control/Model Proces10/Rezervor ==
  q : Inport
  Fcn : Fcn  Expr=sqrt(u)*9
  Gain : Gain  Gain=1/332.5
  Integrator : Integrator  InitialCondition=10.51
  Sum : Sum  Inputs=|+-
  h : Outport
  wires:
  Gain/1 -> Integrator/1
  Fcn/1 -> Sum/2
  Integrator/1 -> h/1, Fcn/1
  Sum/1 -> Gain/1
  q/1 -> Sum/1

== system PI_Level_Control/Model Proces11/Amplificator ==
  ua : Inport
  Constant : Constant  Value=8.1
  Gain : Gain  Gain=2.2
  Gain1 : Gain  Gain=2.2
  Gain2 : Gain  Gain=5
  Saturation : Saturate  UpperLimit=22  LowerLimit=0
  Sum : Sum  Inputs=|+-
  Sum1 : Sum  Inputs=|++
  Switch : Switch  Threshold=8.1  SaturateOnIntegerOverflow=off  InputSameDT=off
  um : Outport
  wires:
  ua/1 -> Gain/1, Sum/1, Gain1/1, Switch/2
  Gain1/1 -> Sum1/1
  Gain/1 -> Switch/3
  Sum1/1 -> Switch/1
  Gain2/1 -> Sum1/2
  Constant/1 -> Sum/2
  Switch/1 -> Saturation/1
  Sum/1 -> Gain2/1
  Saturation/1 -> um/1

== system PI_Level_Control/Model Proces11/Curent Rotoric ==
  h : Inport
  q : Inport  Port=2
  eta : Inport  Port=3
  um : Inport  Port=4
  Constant : Constant  Value=000.1
  Divide : Product  Inputs=**/
  Gain : Gain  Gain=2
  Gain1 : Gain  Gain=k
  Gain2 : Gain  Gain=1e+4
  Product : Product
  Product1 : Product
  Subtract : Sum
  Subtract1 : Sum
  im : Outport
  wires:
  Divide/1 -> im/1
  Subtract1/1 -> Divide/3
  Constant/1 -> Subtract1/1
  Gain2/1 -> Product1/1
  q/1 -> Divide/2, Product/1, Gain1/1
  Subtract/1 -> Divide/1
  Product/1 -> Subtract/2
  Gain/1 -> Subtract/1
  Gain1/1 -> Product/2
  Product1/1 -> Subtract1/2
  um/1 -> Product1/2
  h/1 -> Gain/1
  eta/1 -> Gain2/1

== system PI_Level_Control/Model Proces11/Filtru ==
  q : Inport
  Integrator : Integrator  InitialCondition=27.3
  Sum : Sum  Inputs=|+-
  q_f : Outport
  wires:
  Sum/1 -> Integrator/1
  Integrator/1 -> q_f/1, Sum/2
  q/1 -> Sum/1

== system PI_Level_Control/Model Proces11/Motor ==
  um : Inport
  im : Inport  Port=2
  Add : Sum  Inputs=+-
  Rm : Gain  Gain=3
  kn : Outport
  wires:
  Rm/1 -> Add/2
  um/1 -> Add/1
  im/1 -> Rm/1
  Add/1 -> kn/1

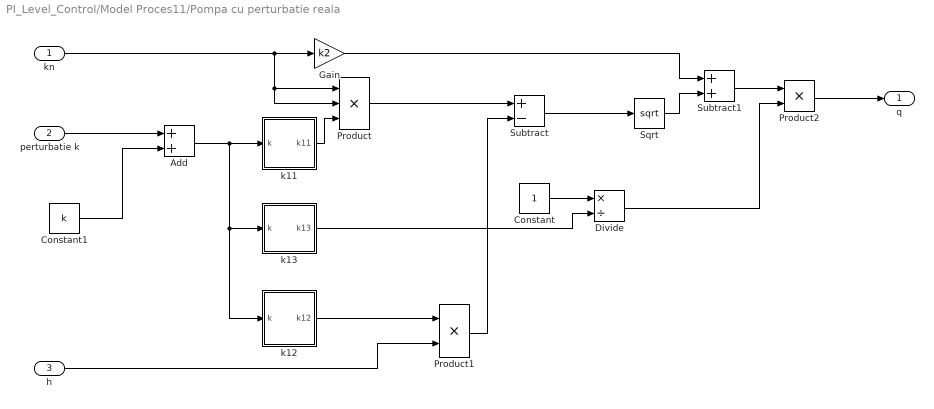
== system PI_Level_Control/Model Proces11/Pompa cu perturbatie reala ==
  kn : Inport
  perturbatie k : Inport  Port=2
  h : Inport  Port=3
  Add : Sum
  Constant : Constant
  Constant1 : Constant  Value=k
  Divide : Product  Inputs=*/
  Gain : Gain  Gain=k2
  Product : Product  Inputs=3
  Product1 : Product
  Product2 : Product
  Sqrt : Sqrt
  Subtract : Sum  Inputs=+-
  Subtract1 : Sum
  k11 : Subsystem
  k12 : Subsystem
  k13 : Subsystem
  q : Outport
  wires:
  h/1 -> Product1/2
  k12/1(k12) -> Product1/1
  Constant1/1 -> Add/2
  Add/1 -> k12/1(k), k13/1(k), k11/1(k)
  Gain/1 -> Subtract1/1
  Product/1 -> Subtract/1
  Divide/1 -> Product2/2
  kn/1 -> Product/2, Product/1, Gain/1
  Subtract/1 -> Sqrt/1
  k13/1(k13) -> Divide/2
  Subtract1/1 -> Product2/1
  k11/1(k11) -> Product/3
  Constant/1 -> Divide/1
  Product1/1 -> Subtract/2
  Sqrt/1 -> Subtract1/2
  perturbatie k/1 -> Add/1
  Product2/1 -> q/1

== system PI_Level_Control/Model Proces11/Randament Pompa ==
  q : Inport
  um : Inport  Port=2
  Gain : Gain  Gain=keta
  Product : Product
  eta : Outport
  wires:
  Gain/1 -> Product/2
  Product/1 -> eta/1
  q/1 -> Product/1
  um/1 -> Gain/1

== system PI_Level_Control/Model Proces11/Rezervor1 ==
  q : Inport
  Fcn : Fcn  Expr=sqrt(u)*6.8
  Gain : Gain  Gain=1/332.5
  Integrator : Integrator  InitialCondition=16.02
  Sum : Sum  Inputs=|+-
  h : Outport
  wires:
  Gain/1 -> Integrator/1
  Fcn/1 -> Sum/2
  Integrator/1 -> h/1, Fcn/1
  Sum/1 -> Gain/1
  q/1 -> Sum/1

== system PI_Level_Control/Model Proces12/Amplificator ==
  ua : Inport
  Constant : Constant  Value=8.1
  Gain : Gain  Gain=2.2
  Gain1 : Gain  Gain=2.2
  Gain2 : Gain  Gain=5
  Saturation : Saturate  UpperLimit=22  LowerLimit=0
  Sum : Sum  Inputs=|+-
  Sum1 : Sum  Inputs=|++
  Switch : Switch  Threshold=8.1  SaturateOnIntegerOverflow=off  InputSameDT=off
  um : Outport
  wires:
  ua/1 -> Gain/1, Sum/1, Gain1/1, Switch/2
  Gain1/1 -> Sum1/1
  Gain/1 -> Switch/3
  Sum1/1 -> Switch/1
  Gain2/1 -> Sum1/2
  Constant/1 -> Sum/2
  Switch/1 -> Saturation/1
  Sum/1 -> Gain2/1
  Saturation/1 -> um/1

== system PI_Level_Control/Model Proces12/Curent Rotoric ==
  h : Inport
  q : Inport  Port=2
  eta : Inport  Port=3
  um : Inport  Port=4
  Constant : Constant  Value=000.1
  Divide : Product  Inputs=**/
  Gain : Gain  Gain=2
  Gain1 : Gain  Gain=k
  Gain2 : Gain  Gain=1e+4
  Product : Product
  Product1 : Product
  Subtract : Sum
  Subtract1 : Sum
  im : Outport
  wires:
  Divide/1 -> im/1
  Subtract1/1 -> Divide/3
  Constant/1 -> Subtract1/1
  Gain2/1 -> Product1/1
  q/1 -> Divide/2, Product/1, Gain1/1
  Subtract/1 -> Divide/1
  Product/1 -> Subtract/2
  Gain/1 -> Subtract/1
  Gain1/1 -> Product/2
  Product1/1 -> Subtract1/2
  um/1 -> Product1/2
  h/1 -> Gain/1
  eta/1 -> Gain2/1

== system PI_Level_Control/Model Proces12/Filtru ==
  q : Inport
  Integrator : Integrator  InitialCondition=29.18
  Sum : Sum  Inputs=|+-
  q_f : Outport
  wires:
  Sum/1 -> Integrator/1
  Integrator/1 -> q_f/1, Sum/2
  q/1 -> Sum/1

== system PI_Level_Control/Model Proces12/Motor ==
  um : Inport
  im : Inport  Port=2
  Add : Sum  Inputs=+-
  Rm : Gain  Gain=3
  kn : Outport
  wires:
  Rm/1 -> Add/2
  um/1 -> Add/1
  im/1 -> Rm/1
  Add/1 -> kn/1

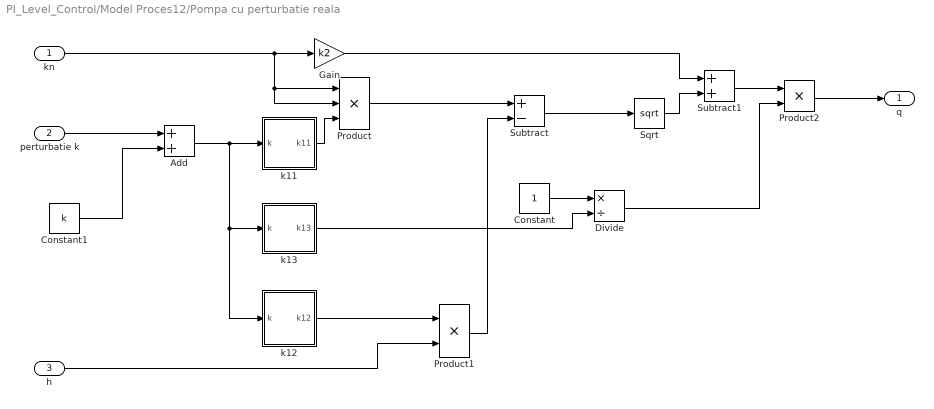
== system PI_Level_Control/Model Proces12/Pompa cu perturbatie reala ==
  kn : Inport
  perturbatie k : Inport  Port=2
  h : Inport  Port=3
  Add : Sum
  Constant : Constant
  Constant1 : Constant  Value=k
  Divide : Product  Inputs=*/
  Gain : Gain  Gain=k2
  Product : Product  Inputs=3
  Product1 : Product
  Product2 : Product
  Sqrt : Sqrt
  Subtract : Sum  Inputs=+-
  Subtract1 : Sum
  k11 : Subsystem
  k12 : Subsystem
  k13 : Subsystem
  q : Outport
  wires:
  h/1 -> Product1/2
  k12/1(k12) -> Product1/1
  Constant1/1 -> Add/2
  Add/1 -> k12/1(k), k13/1(k), k11/1(k)
  Gain/1 -> Subtract1/1
  Product/1 -> Subtract/1
  Divide/1 -> Product2/2
  kn/1 -> Product/2, Product/1, Gain/1
  Subtract/1 -> Sqrt/1
  k13/1(k13) -> Divide/2
  Subtract1/1 -> Product2/1
  k11/1(k11) -> Product/3
  Constant/1 -> Divide/1
  Product1/1 -> Subtract/2
  Sqrt/1 -> Subtract1/2
  perturbatie k/1 -> Add/1
  Product2/1 -> q/1

== system PI_Level_Control/Model Proces12/Randament Pompa ==
  q : Inport
  um : Inport  Port=2
  Gain : Gain  Gain=keta
  Product : Product
  eta : Outport
  wires:
  Gain/1 -> Product/2
  Product/1 -> eta/1
  q/1 -> Product/1
  um/1 -> Gain/1

== system PI_Level_Control/Model Proces12/Rezervor ==
  q : Inport
  Add : Sum
  Constant : Constant  Value=C
  Gain : Gain  Gain=1/332.5
  Integrator : Integrator  InitialCondition=10.51
  Product : Product
  Product1 : Product
  Scope : Scope
  Sqrt : Sqrt
  Step : Step  Time=400  After=2  SampleTime=0
  Sum : Sum  Inputs=|+-
  h : Outport
  perturbatie : Outport  Port=2
  wires:
  Gain/1 -> Integrator/1
  Integrator/1 -> Sqrt/1, h/1
  Sum/1 -> Gain/1
  q/1 -> Sum/1
  Sqrt/1 -> Product1/1, Product/1
  Product/1 -> Scope/1, Sum/2
  Step/1 -> Product1/2, Add/1
  Constant/1 -> Add/2
  Add/1 -> Product/2
  Product1/1 -> perturbatie/1

== system PI_Level_Control/Model Proces13/Amplificator ==
  ua : Inport
  Constant : Constant  Value=8.1
  Gain : Gain  Gain=2.2
  Gain1 : Gain  Gain=2.2
  Gain2 : Gain  Gain=5
  Saturation : Saturate  UpperLimit=22  LowerLimit=0
  Sum : Sum  Inputs=|+-
  Sum1 : Sum  Inputs=|++
  Switch : Switch  Threshold=8.1  SaturateOnIntegerOverflow=off  InputSameDT=off
  um : Outport
  wires:
  ua/1 -> Gain/1, Sum/1, Gain1/1, Switch/2
  Gain1/1 -> Sum1/1
  Gain/1 -> Switch/3
  Sum1/1 -> Switch/1
  Gain2/1 -> Sum1/2
  Constant/1 -> Sum/2
  Switch/1 -> Saturation/1
  Sum/1 -> Gain2/1
  Saturation/1 -> um/1

== system PI_Level_Control/Model Proces13/Curent Rotoric ==
  h : Inport
  q : Inport  Port=2
  eta : Inport  Port=3
  um : Inport  Port=4
  Constant : Constant  Value=000.1
  Divide : Product  Inputs=**/
  Gain : Gain  Gain=2
  Gain1 : Gain  Gain=k
  Gain2 : Gain  Gain=1e+4
  Product : Product
  Product1 : Product
  Subtract : Sum
  Subtract1 : Sum
  im : Outport
  wires:
  Divide/1 -> im/1
  Subtract1/1 -> Divide/3
  Constant/1 -> Subtract1/1
  Gain2/1 -> Product1/1
  q/1 -> Divide/2, Product/1, Gain1/1
  Subtract/1 -> Divide/1
  Product/1 -> Subtract/2
  Gain/1 -> Subtract/1
  Gain1/1 -> Product/2
  Product1/1 -> Subtract1/2
  um/1 -> Product1/2
  h/1 -> Gain/1
  eta/1 -> Gain2/1

== system PI_Level_Control/Model Proces13/Filtru ==
  q : Inport
  Integrator : Integrator  InitialCondition=27.3
  Sum : Sum  Inputs=|+-
  q_f : Outport
  wires:
  Sum/1 -> Integrator/1
  Integrator/1 -> q_f/1, Sum/2
  q/1 -> Sum/1

== system PI_Level_Control/Model Proces13/Motor ==
  um : Inport
  im : Inport  Port=2
  Add : Sum  Inputs=+-
  Rm : Gain  Gain=3
  kn : Outport
  wires:
  Rm/1 -> Add/2
  um/1 -> Add/1
  im/1 -> Rm/1
  Add/1 -> kn/1

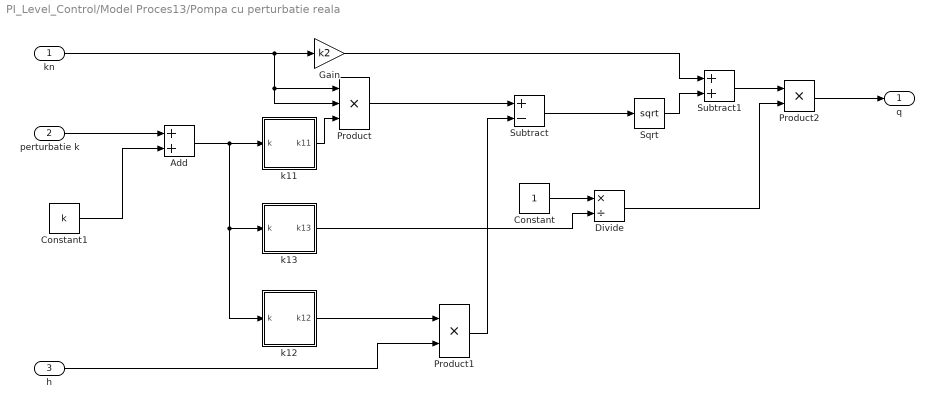
== system PI_Level_Control/Model Proces13/Pompa cu perturbatie reala ==
  kn : Inport
  perturbatie k : Inport  Port=2
  h : Inport  Port=3
  Add : Sum
  Constant : Constant
  Constant1 : Constant  Value=k
  Divide : Product  Inputs=*/
  Gain : Gain  Gain=k2
  Product : Product  Inputs=3
  Product1 : Product
  Product2 : Product
  Sqrt : Sqrt
  Subtract : Sum  Inputs=+-
  Subtract1 : Sum
  k11 : Subsystem
  k12 : Subsystem
  k13 : Subsystem
  q : Outport
  wires:
  h/1 -> Product1/2
  k12/1(k12) -> Product1/1
  Constant1/1 -> Add/2
  Add/1 -> k12/1(k), k13/1(k), k11/1(k)
  Gain/1 -> Subtract1/1
  Product/1 -> Subtract/1
  Divide/1 -> Product2/2
  kn/1 -> Product/2, Product/1, Gain/1
  Subtract/1 -> Sqrt/1
  k13/1(k13) -> Divide/2
  Subtract1/1 -> Product2/1
  k11/1(k11) -> Product/3
  Constant/1 -> Divide/1
  Product1/1 -> Subtract/2
  Sqrt/1 -> Subtract1/2
  perturbatie k/1 -> Add/1
  Product2/1 -> q/1

== system PI_Level_Control/Model Proces13/Randament Pompa ==
  q : Inport
  um : Inport  Port=2
  Gain : Gain  Gain=keta
  Product : Product
  eta : Outport
  wires:
  Gain/1 -> Product/2
  Product/1 -> eta/1
  q/1 -> Product/1
  um/1 -> Gain/1

== system PI_Level_Control/Model Proces13/Rezervor ==
  q : Inport
  Add : Sum
  Constant : Constant  Value=C
  Gain : Gain  Gain=1/332.5
  Integrator : Integrator  InitialCondition=16.02
  Product : Product
  Product1 : Product
  Scope : Scope
  Sqrt : Sqrt
  Step : Step  Time=550  After=2  SampleTime=0
  Sum : Sum  Inputs=|+-
  h : Outport
  perturbatie : Outport  Port=2
  wires:
  Gain/1 -> Integrator/1
  Integrator/1 -> Sqrt/1, h/1
  Sum/1 -> Gain/1
  q/1 -> Sum/1
  Sqrt/1 -> Product1/1, Product/1
  Product/1 -> Scope/1, Sum/2
  Step/1 -> Product1/2, Add/1
  Constant/1 -> Add/2
  Add/1 -> Product/2
  Product1/1 -> perturbatie/1

== system PI_Level_Control/Model Proces2/Amplificator ==
  ua : Inport
  Constant : Constant  Value=8.1
  Gain : Gain  Gain=2.2
  Gain1 : Gain  Gain=2.2
  Gain2 : Gain  Gain=5
  Saturation : Saturate  UpperLimit=22  LowerLimit=0
  Sum : Sum  Inputs=|+-
  Sum1 : Sum  Inputs=|++
  Switch : Switch  Threshold=8.1  SaturateOnIntegerOverflow=off  InputSameDT=off
  um : Outport
  wires:
  ua/1 -> Gain/1, Sum/1, Gain1/1, Switch/2
  Gain1/1 -> Sum1/1
  Gain/1 -> Switch/3
  Sum1/1 -> Switch/1
  Gain2/1 -> Sum1/2
  Constant/1 -> Sum/2
  Switch/1 -> Saturation/1
  Sum/1 -> Gain2/1
  Saturation/1 -> um/1

== system PI_Level_Control/Model Proces2/Curent Rotoric ==
  h : Inport
  q : Inport  Port=2
  eta : Inport  Port=3
  um : Inport  Port=4
  Constant : Constant  Value=000.1
  Divide : Product  Inputs=**/
  Gain : Gain  Gain=2
  Gain1 : Gain  Gain=k
  Gain2 : Gain  Gain=1e+4
  Product : Product
  Product1 : Product
  Subtract : Sum
  Subtract1 : Sum
  im : Outport
  wires:
  Divide/1 -> im/1
  Subtract1/1 -> Divide/3
  Constant/1 -> Subtract1/1
  Gain2/1 -> Product1/1
  q/1 -> Divide/2, Product/1, Gain1/1
  Subtract/1 -> Divide/1
  Product/1 -> Subtract/2
  Gain/1 -> Subtract/1
  Gain1/1 -> Product/2
  Product1/1 -> Subtract1/2
  um/1 -> Product1/2
  h/1 -> Gain/1
  eta/1 -> Gain2/1

== system PI_Level_Control/Model Proces2/Filtru ==
  q : Inport
  Integrator : Integrator  InitialCondition=27.3
  Sum : Sum  Inputs=|+-
  q_f : Outport
  wires:
  Sum/1 -> Integrator/1
  Integrator/1 -> q_f/1, Sum/2
  q/1 -> Sum/1

== system PI_Level_Control/Model Proces2/Motor ==
  um : Inport
  im : Inport  Port=2
  Add : Sum  Inputs=+-
  Rm : Gain  Gain=3
  kn : Outport
  wires:
  Rm/1 -> Add/2
  um/1 -> Add/1
  im/1 -> Rm/1
  Add/1 -> kn/1

== system PI_Level_Control/Model Proces2/Pompa ==
  kn : Inport
  h : Inport  Port=2
  Gain : Gain  Gain=k2
  Gain1 : Gain  Gain=k11
  Gain2 : Gain  Gain=k12
  Gain3 : Gain  Gain=1/k13
  Product : Product
  Sqrt : Sqrt
  Subtract : Sum  Inputs=+-
  Subtract1 : Sum
  q : Outport
  wires:
  Gain1/1 -> Subtract/1
  Gain2/1 -> Subtract/2
  Product/1 -> Gain1/1
  Gain/1 -> Subtract1/1
  kn/1 -> Product/2, Product/1, Gain/1
  Subtract/1 -> Sqrt/1
  Subtract1/1 -> Gain3/1
  Sqrt/1 -> Subtract1/2
  Gain3/1 -> q/1
  h/1 -> Gain2/1

== system PI_Level_Control/Model Proces2/Randament Pompa ==
  q : Inport
  um : Inport  Port=2
  Gain : Gain  Gain=keta
  Product : Product
  eta : Outport
  wires:
  Gain/1 -> Product/2
  Product/1 -> eta/1
  q/1 -> Product/1
  um/1 -> Gain/1

== system PI_Level_Control/Model Proces2/Rezervor ==
  q : Inport
  Fcn : Fcn  Expr=sqrt(u)*6.8
  Gain : Gain  Gain=1/332.5
  Integrator : Integrator  InitialCondition=16.02
  Sum : Sum  Inputs=|+-
  h : Outport
  wires:
  Gain/1 -> Integrator/1
  Fcn/1 -> Sum/2
  Integrator/1 -> h/1, Fcn/1
  Sum/1 -> Gain/1
  q/1 -> Sum/1

== system PI_Level_Control/Model Proces3/Amplificator ==
  ua : Inport
  Constant : Constant  Value=8.1
  Gain : Gain  Gain=2.2
  Gain1 : Gain  Gain=2.2
  Gain2 : Gain  Gain=5
  Saturation : Saturate  UpperLimit=22  LowerLimit=0
  Sum : Sum  Inputs=|+-
  Sum1 : Sum  Inputs=|++
  Switch : Switch  Threshold=8.1  SaturateOnIntegerOverflow=off  InputSameDT=off
  um : Outport
  wires:
  ua/1 -> Gain/1, Sum/1, Gain1/1, Switch/2
  Gain1/1 -> Sum1/1
  Gain/1 -> Switch/3
  Sum1/1 -> Switch/1
  Gain2/1 -> Sum1/2
  Constant/1 -> Sum/2
  Switch/1 -> Saturation/1
  Sum/1 -> Gain2/1
  Saturation/1 -> um/1

== system PI_Level_Control/Model Proces3/Curent Rotoric ==
  h : Inport
  q : Inport  Port=2
  eta : Inport  Port=3
  um : Inport  Port=4
  Constant : Constant  Value=000.1
  Divide : Product  Inputs=**/
  Gain : Gain  Gain=2
  Gain1 : Gain  Gain=k
  Gain2 : Gain  Gain=1e+4
  Product : Product
  Product1 : Product
  Subtract : Sum
  Subtract1 : Sum
  im : Outport
  wires:
  Divide/1 -> im/1
  Subtract1/1 -> Divide/3
  Constant/1 -> Subtract1/1
  Gain2/1 -> Product1/1
  q/1 -> Divide/2, Product/1, Gain1/1
  Subtract/1 -> Divide/1
  Product/1 -> Subtract/2
  Gain/1 -> Subtract/1
  Gain1/1 -> Product/2
  Product1/1 -> Subtract1/2
  um/1 -> Product1/2
  h/1 -> Gain/1
  eta/1 -> Gain2/1

== system PI_Level_Control/Model Proces3/Filtru ==
  q : Inport
  Integrator : Integrator  InitialCondition=29.18
  Sum : Sum  Inputs=|+-
  q_f : Outport
  wires:
  Sum/1 -> Integrator/1
  Integrator/1 -> q_f/1, Sum/2
  q/1 -> Sum/1
